simulink model "StateSpaceLinearR2019a"  (R2019a)
settings: Solver=FixedStepAuto  StartTime=0.0  StopTime=inf  RelTol=1e-3  EnableMultiTasking=on
libraries: arduinolib x7, simulink x1
settings Model: SimulationMode=external  ExtModeTrigDuration=2  Creator=Win7  LastModifiedBy=manh
settings DataIOCC: SaveFormat=Array  SaveOutput=off  SaveTime=off  ReturnWorkspaceOutputs=off
settings OptimizationCC: PassReuseOutputArgsAs=Individual arguments  MaxStackSize=64
settings DebuggingCC: ParameterTunabilityLossMsg=error  ArithmeticOperatorsInVariantConditions=warning
settings HardwareCC: ProdBitPerInt=16  ProdBitPerPointer=16  ProdBitPerSizeT=16  ProdBitPerPtrDiffT=16  ProdLargestAtomicFloat=None  ProdWordSize=8  ProdHWDeviceType=Atmel->AVR
settings SFSimCC: SimUseLocalCustomCode=off  MATLABDynamicMemAlloc=off
settings RTWCC: SystemTargetFile=ert.tlc  HardwareBoard=Arduino Mega 2560  TLCOptions=-aInlineSetEventsForThisBaseRateFcn=TLC_FALSE -aSuppressMultiTaskScheduler=TLC_FALSE -aRateBasedStepFcn=1  TemplateMakefile=ert_default_tmf  GenerateReport=on  RTWUseLocalCustomCode=off  Toolchain=Arduino AVR  BuildConfiguration=Faster Runs  IncludeHyperlinkInReport=on  LaunchReport=on  GenerateTraceInfo=on  GenerateTraceReport=on  GenerateTraceReportSl=on  GenerateTraceReportSf=on  GenerateTraceReportEml=on
settings CodeAppCC: ForceParamTrailComments=on  IgnoreCustomStorageClasses=off  OperatorAnnotations=on  SimulinkDataObjDesc=on  SFDataObjDesc=on  InsertBlockDesc=on
settings ERTTargetCC: SupportContinuousTime=on  SupportVariableSizeSignals=on

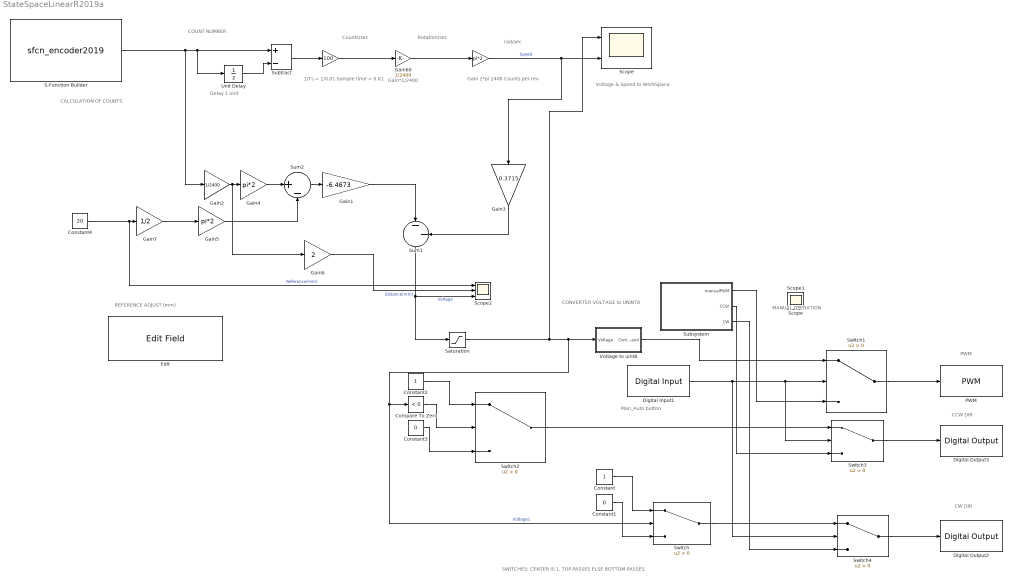
== system StateSpaceLinearR2019a ==
  note: CALCULATION OF COUNTS
  note: SWITCHES: CENTER IS 1, TOP PASSES ELSE BOTTOM PASSES
  note: CONVERTER
      | VOLTAGE to UNINT8
  note: MANUAL OPERATION
  note: Voltage & Speed
      | to WorkSpace
  note: Gain 2*pi
      | 2400 Counts per rev
  note: 1/Ts = 1/0.01
      | Sample time = 0.01
  note: Counts/sec
  note: Delay 1 unit
  note: CW DIR
  note: CCW DIR
  note: PWM
  note: Man_Auto button
  note: Rotation/sec
  note: rad/sec
  note: Gain*1/2400
  note: COUNT NUMBER
  note: REFERENCE ADJUST (mm)
  " " : Gain  Gain=100  OutDataTypeStr=double
  " " : Gain  Gain=pi*2  OutDataTypeStr=double
  Compare To Zero : simulink/Logic and Bit Operations/Compare To Zero  relop=<  OutDataTypeStr=boolean
  Constant : Constant
  Constant1 : Constant  Value=0
  Constant2 : Constant
  Constant3 : Constant  Value=0
  Constant4 : Constant  Value=20
  Digital Input1 : arduinolib/Digital Input  pinNumber=28  sampleTime=0.01  blockPlatform=arduino
      settings: SourceProductName=Simulink Support Package for Arduino Hardware
  Digital Output2 : arduinolib/Digital Output  pinNumber=36  blockPlatform=arduino
  Digital Output3 : arduinolib/Digital Output  pinNumber=38  blockPlatform=arduino
  Edit : EditField  LabelPosition=Hide  Alignment=Center
  Gain1 : Gain  Gain=-6.4673
  Gain2 : Gain  Gain=1/2400  ParamDataTypeStr=double  OutDataTypeStr=double
  Gain3 : Gain  Gain=0.3715
  Gain4 : Gain  Gain=pi*2  ParamDataTypeStr=double  OutDataTypeStr=double
  Gain5 : Gain  Gain=pi*2  ParamDataTypeStr=double  OutDataTypeStr=double
  Gain6 : Gain  Gain=2  ParamDataTypeStr=double  OutDataTypeStr=double
  Gain60 : Gain  Gain=1/2400  OutDataTypeStr=double
  Gain7 : Gain  Gain=1/2  ParamDataTypeStr=double  OutDataTypeStr=double
  PWM : arduinolib/PWM  pinNumber=7  EnableInputFrequency=off  InitialFrequency=2000  InitialDutyCycle=0  NotificationType=None  blockPlatform=arduino
  S-Function Builder : S-Function  FunctionName=sfcn_encoder2019  Parameters=uint8(0),uint8(2),uint8(3)  SFunctionModules=sfcn_encoder2019_wrapper  SFunctionDeploymentMode=off  EnableBusSupport=off  mask(S-Function Builder){}
      mask help: Simulink:masks:SFunctionBuilder_MD
      mask init:
      | val = [[.9  0.75 0.75 1 1 .9 .9 1]',[1 1 0.75 0.75 .9 .9 1 .9]'];try , sys = get_param(gcb,'SfunBuilderFcnName');if isempty(sys), sys = get_param(gcb,'FunctionName'); end,catch, sys = get_param(gcb,'FunctionName'); end
      settings: CopyFcn=set_param(gcbh,'LinkStatus','none')  PreSaveFcn=try, set_param(gcb,'FunctionName','sfcn_encoder2019'), end  OpenFcn=sfunctionwizard(gcbh)
      mask Display: plot(val(:,1),val(:,2)),disp(sys), port_label('output',1,'pos')
  Saturation : Saturate  UpperLimit=12  LowerLimit=-12
  "Scope " : Scope  NumInputPorts=2
  Scope2 : Scope  NumInputPorts=3
  Subsystem : Subsystem
  Subtract : Sum  Inputs=+-
  Sum1 : Sum  Inputs=|--
  Sum2 : Sum  Inputs=|+-
  Switch{,1..4} (5 alike) : Switch  Criteria=u2 > Threshold
  Unit Delay : UnitDelay  SampleTime=-1  HasFrameUpgradeWarning=on
  Voltage to uint8 : Subsystem
  Scope : Scope
  Scope1 : Scope
  wires:
  Saturation/1 -> "Scope "/1, Switch/2, Compare To Zero/1, Voltage to uint8/1(Voltage)  "Voltage1"
  Compare To Zero/1 -> Switch2/2
  Constant/1 -> Switch/1
  Constant1/1 -> Switch/3
  Constant2/1 -> Switch2/1
  Constant3/1 -> Switch2/3
  Digital Input1/1 -> Switch1/2, Switch3/2, Switch4/2
  Voltage to uint8/1(Command) -> Switch1/1
  Switch2/1 -> Switch3/1
  Switch/1 -> Switch4/1
  Subsystem/1(manualPWM) -> Switch1/3
  Subsystem/2(CCW) -> Switch3/3
  Subsystem/3(CW) -> Switch4/3
  Switch3/1 -> Digital Output3/1
  Switch4/1 -> Digital Output2/1
  Switch1/1 -> PWM/1
  Unit Delay/1 -> Subtract/2
  Gain60/1 -> " "/1
  " "/1 -> Gain3/1, "Scope "/2  "Speed"
  Subtract/1 -> " "/1
  " "/1 -> Gain60/1
  Gain6/1 -> Scope2/2  "Distance(mm)"
  Gain5/1 -> Sum2/2
  Gain1/1 -> Sum1/1
  Constant4/1 -> Scope2/1, Gain7/1  "Reference(mm)"
  Gain4/1 -> Sum2/1
  Gain2/1 -> Gain6/1, Gain4/1
  Sum2/1 -> Gain1/1
  Gain3/1 -> Sum1/2
  Sum1/1 -> Scope2/3, Saturation/1  "Voltage"
  Gain7/1 -> Gain5/1
  S-Function Builder/1 -> Gain2/1, Subtract/1, Unit Delay/1

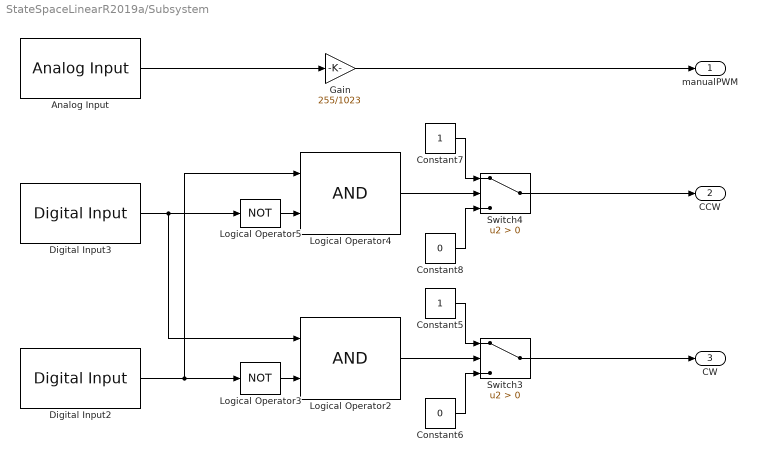
== system StateSpaceLinearR2019a/Subsystem ==
  Analog Input : arduinolib/Analog Input  pinNumber=5  sampleTime=0.01  blockPlatform=arduino
  Constant5 : Constant
  Constant6 : Constant  Value=0
  Constant7 : Constant
  Constant8 : Constant  Value=0
  Digital Input2 : arduinolib/Digital Input  pinNumber=22  sampleTime=0.01  blockPlatform=arduino
      settings: SourceProductName=Simulink Support Package for Arduino Hardware
  Digital Input3 : arduinolib/Digital Input  pinNumber=24  sampleTime=0.01  blockPlatform=arduino
      settings: SourceProductName=Simulink Support Package for Arduino Hardware
  Gain : Gain  Gain=255/1023
  Logical Operator2 : Logic  AllPortsSameDT=off  OutDataTypeStr=boolean
  Logical Operator3 : Logic  Operator=NOT  AllPortsSameDT=off  OutDataTypeStr=boolean
  Logical Operator4 : Logic  AllPortsSameDT=off  OutDataTypeStr=boolean
  Logical Operator5 : Logic  Operator=NOT  AllPortsSameDT=off  OutDataTypeStr=boolean
  Switch3 : Switch  Criteria=u2 > Threshold
  Switch4 : Switch  Criteria=u2 > Threshold
  manualPWM : Outport
  CCW : Outport  Port=2
  CW : Outport  Port=3
  wires:
  Constant6/1 -> Switch3/3
  Constant7/1 -> Switch4/1
  Logical Operator5/1 -> Logical Operator4/2
  Constant5/1 -> Switch3/1
  Switch3/1 -> CW/1
  Logical Operator3/1 -> Logical Operator2/2
  Logical Operator2/1 -> Switch3/2
  Switch4/1 -> CCW/1
  Digital Input2/1 -> Logical Operator4/1, Logical Operator3/1
  Gain/1 -> manualPWM/1
  Analog Input/1 -> Gain/1
  Logical Operator4/1 -> Switch4/2
  Digital Input3/1 -> Logical Operator5/1, Logical Operator2/1
  Constant8/1 -> Switch4/3

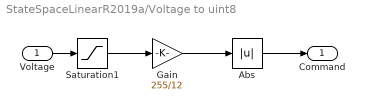
== system StateSpaceLinearR2019a/Voltage to uint8 ==
  Voltage : Inport
  Abs : Abs  OutDataTypeStr=uint8
  Gain : Gain  Gain=255/12  OutDataTypeStr=single
  Saturation1 : Saturate  UpperLimit=12  LowerLimit=-12
  Command : Outport
  wires:
  Voltage/1 -> Saturation1/1
  Saturation1/1 -> Gain/1
  Gain/1 -> Abs/1
  Abs/1 -> Command/1
